simulink model "collector"  (R2018a)
settings: Solver=FixedStepAuto  StartTime=0.0  StopTime=20  FixedStep=0.01  RelTol=1e-3
undefined symbols (not defined in the file): sigbuilder_block
settings Model: EnablePacing=on  Creator=U500304  LastModifiedBy=U500304
settings SolverCC: ZeroCrossAlgorithm=Adaptive
settings DataIOCC: SaveOutput=off  SaveTime=off
settings DebuggingCC: MaxConsecutiveZCsMsg=none

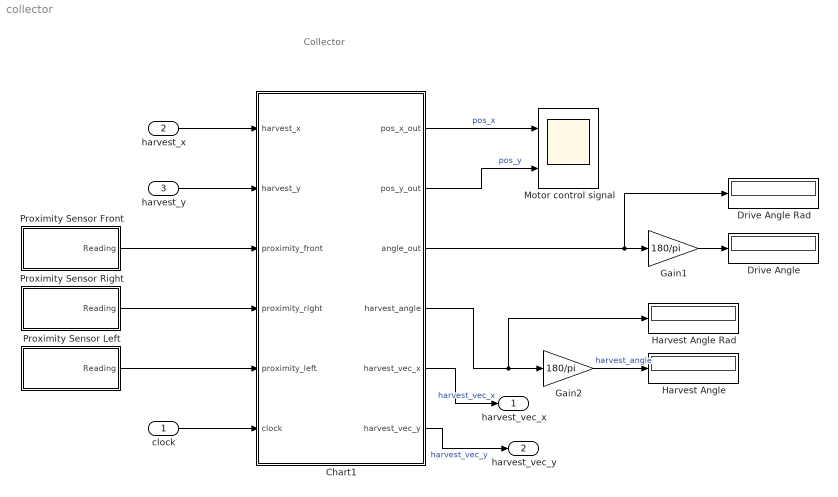
== system collector ==
  note: Collector
  clock : Inport  OutDataTypeStr=double  PortDimensions=1  SampleTime=0
  harvest_x : Inport  Port=2  OutDataTypeStr=double  PortDimensions=1  SampleTime=0
  harvest_y : Inport  Port=3  OutDataTypeStr=double  PortDimensions=1  SampleTime=0
  Chart1 : Stateflow chart  TreatAsAtomicUnit=on
  Drive Angle : Display
  Drive Angle Rad : Display
  Gain1 : Gain  Gain=180/pi
  Gain2 : Gain  Gain=180/pi
  Harvest Angle : Display
  Harvest Angle Rad : Display
  Motor control signal : Scope  NumInputPorts=2
  Proximity Sensor Front : Subsystem  Tag=STV Subsys  LoadFcn=sigbuilder_block('load');  StartFcn=sigbuilder_block('start');  StopFcn=sigbuilder_block('stop');  ClipboardFcn=sigbuilder_block('clipboard');  mask(Sigbuilder block){tuvar=[0:10]}
      mask help: Simulink:masks:SigbuilderBlock_MD
      mask init:
      | if ~strcmp(get_param(bdroot(gcbh),'SimulationStatus'),'stopped') tuvar = sigbuilder_block('maskInit'); end
      settings: CopyFcn=sigbuilder_block('copy');  DeleteFcn=sigbuilder_block('delete');  ModelCloseFcn=sigbuilder_block('modelClose');  PreSaveFcn=sigbuilder_block('preSave');  PauseFcn=sigbuilder_block('pause');  ContinueFcn=sigbuilder_block('continue');  NameChangeFcn=sigbuilder_block('namechange');  OpenFcn=sigbuilder_block('open',[5.4 30 1141.2 522.6 ]);  CloseFcn=sigbuilder_block('close');
      mask Display: plot(0, 0, 100, 100,[2, 2, 32, 32, 2], [68, 8, 8, 68, 68],[32, 2], [38, 38], [32, 19, 2],[53, 60, 44], [32, 17, 17, 2],[16, 16, 31, 31]);txt = getActiveGroup(gcbh);text(2, 100, txt,'verticalAlignment', 'top');
  Proximity Sensor Left : Subsystem  Tag=STV Subsys  LoadFcn=sigbuilder_block('load');  StartFcn=sigbuilder_block('start');  StopFcn=sigbuilder_block('stop');  ClipboardFcn=sigbuilder_block('clipboard');  mask(Sigbuilder block){tuvar=[0:10]}
      mask help: Simulink:masks:SigbuilderBlock_MD
      mask init:
      | if ~strcmp(get_param(bdroot(gcbh),'SimulationStatus'),'stopped') tuvar = sigbuilder_block('maskInit'); end
      settings: CopyFcn=sigbuilder_block('copy');  DeleteFcn=sigbuilder_block('delete');  ModelCloseFcn=sigbuilder_block('modelClose');  PreSaveFcn=sigbuilder_block('preSave');  PauseFcn=sigbuilder_block('pause');  ContinueFcn=sigbuilder_block('continue');  NameChangeFcn=sigbuilder_block('namechange');  OpenFcn=sigbuilder_block('open',[5.4 30 1141.2 522.6 ]);  CloseFcn=sigbuilder_block('close');
      mask Display: plot(0, 0, 100, 100,[2, 2, 32, 32, 2], [68, 8, 8, 68, 68],[32, 2], [38, 38], [32, 19, 2],[53, 60, 44], [32, 17, 17, 2],[16, 16, 31, 31]);txt = getActiveGroup(gcbh);text(2, 100, txt,'verticalAlignment', 'top');
  Proximity Sensor Right : Subsystem  Tag=STV Subsys  LoadFcn=sigbuilder_block('load');  StartFcn=sigbuilder_block('start');  StopFcn=sigbuilder_block('stop');  ClipboardFcn=sigbuilder_block('clipboard');  mask(Sigbuilder block){tuvar=[0:10]}
      mask help: Simulink:masks:SigbuilderBlock_MD
      mask init:
      | if ~strcmp(get_param(bdroot(gcbh),'SimulationStatus'),'stopped') tuvar = sigbuilder_block('maskInit'); end
      settings: CopyFcn=sigbuilder_block('copy');  DeleteFcn=sigbuilder_block('delete');  ModelCloseFcn=sigbuilder_block('modelClose');  PreSaveFcn=sigbuilder_block('preSave');  PauseFcn=sigbuilder_block('pause');  ContinueFcn=sigbuilder_block('continue');  NameChangeFcn=sigbuilder_block('namechange');  OpenFcn=sigbuilder_block('open',[5.4 30 1141.2 522.6 ]);  CloseFcn=sigbuilder_block('close');
      mask Display: plot(0, 0, 100, 100,[2, 2, 32, 32, 2], [68, 8, 8, 68, 68],[32, 2], [38, 38], [32, 19, 2],[53, 60, 44], [32, 17, 17, 2],[16, 16, 31, 31]);txt = getActiveGroup(gcbh);text(2, 100, txt,'verticalAlignment', 'top');
  harvest_vec_x : Outport  OutDataTypeStr=double  PortDimensions=1  SampleTime=0
  harvest_vec_y : Outport  Port=2  OutDataTypeStr=double  PortDimensions=1  SampleTime=0
  wires:
  Proximity Sensor Right/1(Reading) -> Chart1/4(proximity_right)
  Chart1/1(pos_x_out) -> Motor control signal/1  "pos_x"
  Chart1/3(angle_out) -> Gain1/1, Drive Angle Rad/1
  Proximity Sensor Left/1(Reading) -> Chart1/5(proximity_left)
  Chart1/2(pos_y_out) -> Motor control signal/2  "pos_y"
  Gain1/1 -> Drive Angle/1
  Chart1/4(harvest_angle) -> Harvest Angle Rad/1, Gain2/1
  Proximity Sensor Front/1(Reading) -> Chart1/3(proximity_front)
  Gain2/1 -> Harvest Angle/1  "harvest_angle"
  harvest_x/1 -> Chart1/1(harvest_x)
  clock/1 -> Chart1/6(clock)
  harvest_y/1 -> Chart1/2(harvest_y)
  Chart1/5(harvest_vec_x) -> harvest_vec_x/1  "harvest_vec_x"
  Chart1/6(harvest_vec_y) -> harvest_vec_y/1  "harvest_vec_y"

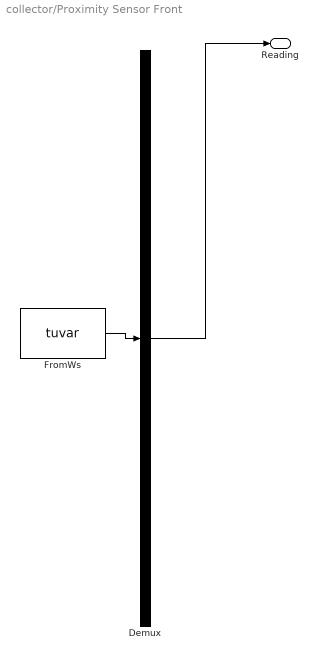
== system collector/Proximity Sensor Front ==
  Demux : Demux  Tag=STV Demux  Outputs=1
  FromWs : FromWorkspace  Tag=STV FromWs  VariableName=tuvar  SampleTime=0
      SigBuilderData=|
      | common.afterFinalStr = 'Extrapolate'
      | common.sampleTime = 0
      | dataSet.timeRange = [0 10]
      | dataSet.name = 'Proximity Front'
      | sbobj.Groups.Name = 'Proximity Front'
      | sbobj.Groups.Signals.Name = 'Reading'
      | sbobj.Groups.Signals.XData = [0 1 4 4 10]
      | sbobj.Groups.Signals.YData = [4.95 4.95 5 4.95 4.9]
  Reading : Outport  Tag=STV Outport
  wires:
  Demux/1 -> Reading/1
  FromWs/1 -> Demux/1

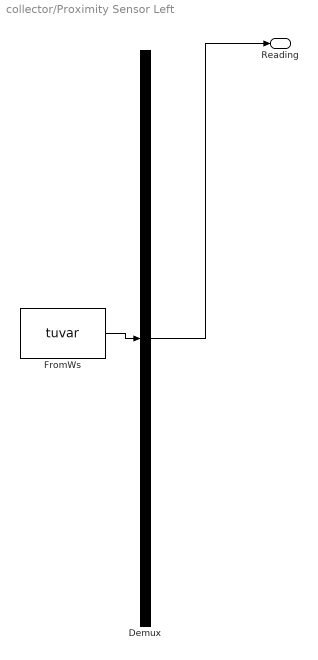
== system collector/Proximity Sensor Left ==
  Demux : Demux  Tag=STV Demux  Outputs=1
  FromWs : FromWorkspace  Tag=STV FromWs  VariableName=tuvar  SampleTime=0
      SigBuilderData=|
      | common.afterFinalStr = 'Extrapolate'
      | common.sampleTime = 0
      | dataSet.timeRange = [0 10]
      | dataSet.name = 'Proximity Left'
      | sbobj.Groups.Name = 'Proximity Left'
      | sbobj.Groups.Signals.Name = 'Reading'
      | sbobj.Groups.Signals.XData = [0 1 4 4 10]
      | sbobj.Groups.Signals.YData = [9 9.05 8.9 8.95 9.7]
  Reading : Outport  Tag=STV Outport
  wires:
  Demux/1 -> Reading/1
  FromWs/1 -> Demux/1

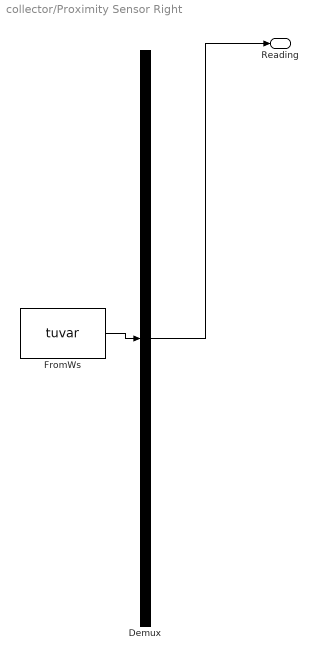
== system collector/Proximity Sensor Right ==
  Demux : Demux  Tag=STV Demux  Outputs=1
  FromWs : FromWorkspace  Tag=STV FromWs  VariableName=tuvar  SampleTime=0
      SigBuilderData=|
      | common.afterFinalStr = 'Extrapolate'
      | common.sampleTime = 0
      | dataSet.timeRange = [0 10]
      | dataSet.name = 'Proximity Right'
      | sbobj.Groups.Name = 'Proximity Right'
      | sbobj.Groups.Signals.Name = 'Reading'
      | sbobj.Groups.Signals.XData = [0 1 10]
      | sbobj.Groups.Signals.YData = [4.6 4.6 4.6]
  Reading : Outport  Tag=STV Outport
  wires:
  FromWs/1 -> Demux/1
  Demux/1 -> Reading/1

== stateflow chart collector/Chart1 ==
  settings: updateMethod=CONTINUOUS
  state Annoy
    state Move
      du:
      pos_x_dot = (r / 2) * (ul + ur) * cos(angle);
      pos_y_dot = (r / 2) * (ul + ur) * sin(angle);
      angle_dot = (r / L) * (ur - ul);
      pos_x_out = pos_x;
      pos_y_out = pos_y;
      angle_out = angle;
    note: Tries to annoy other robots by pushing them using proximity sensor readings
    (default) -> Annoy.Move
    Annoy.Move -> Annoy.Move [order 2] : [proximity_right < proximity_front && turn == 0]
        | {ul = 1; ur = -1; turn = 2;}
    Annoy.Move -> Annoy.Move [order 1] : [proximity_left < proximity_front && turn == 0]
        | {ul = -1; ur = 1; turn = 1;}
    Annoy.Move -> Annoy.Move [order 3] : [(proximity_front < proximity_right && proximity_front < proximity_left) && turn > 0]{ul = 1; ur = 1; turn = 0}
  state Harvest
    state Move
      en:
      harvest_vec_x = (harvest_x - pos_x);
      harvest_vec_y = (harvest_y - pos_y);
      harvest_angle = atan(harvest_vec_y / harvest_vec_x)
      du:
      pos_x_dot = (r / 2) * (ul + ur) * cos(angle);
      pos_y_dot = (r / 2) * (ul + ur) * sin(angle);
      angle_dot = (r / L) * (ur - ul);
      pos_x_out = pos_x;
      pos_y_out = pos_y;
      angle_out = angle;
    state Stop
    note: Drives to the given location of light
    (default) -> Harvest.Move
    Harvest.Move -> Harvest.Move [order 2] : [(angle - harvest_angle > 0.005) && turn == 0]
        | {ul = 1; ur = -1; turn = 2;}
    Harvest.Move -> Stop [order 4] : [abs(harvest_x - pos_x) <= 0.1 && abs(harvest_y - pos_y) <= 0.1]
    Harvest.Move -> Harvest.Move [order 1] : [(angle - harvest_angle < -0.005) && turn == 0]
        | {ul = -1; ur = 1; turn = 1;}
    Harvest.Move -> Harvest.Move [order 3] : [(angle > harvest_angle && turn == 1) || (angle < harvest_angle && turn == 2)]
        | {ul = 1; ur = 1; turn = 0}
  (default) -> Annoy : {
      | pos_x = 0;
      | pos_y = 0'
      | }
  Annoy -> Harvest : [harvest_x > -1 && harvest_y > -1]
  data: harvest_x input; harvest_y input; proximity_front input; proximity_right input; proximity_left input; clock input; pos_x local; pos_y local; pos_x_out output; pos_y_out output; target_dir_x local; target_dir_y local; r constant double =10; L constant double =100; ul local =1; ur local =1; angle local =0; angle_out output; turn local =0; harvest_angle output; harvest_vec_x output; harvest_vec_y output
  data pos_x settings: updateMethod=SF_CONTINUOUS_TIME_DATA
  data pos_y settings: updateMethod=SF_CONTINUOUS_TIME_DATA
  data angle settings: updateMethod=SF_CONTINUOUS_TIME_DATA
